simulink model "problem1"  (R2020a)
settings: Solver=VariableStepAuto  StartTime=0.0  StopTime=10.0  RelTol=1e-3
values from neighbouring files (symbols this model uses):
  b = 50.0    [problem_1data.sldd]
  K1 = 50.0    [problem_1data.sldd]
  K12 = 500.0    [problem_1data.sldd]
  M1 = 100.0    [problem_1data.sldd]
  M2 = 5.0    [problem_1data.sldd]
settings Model: Creator=USER  LastModifiedBy=USER

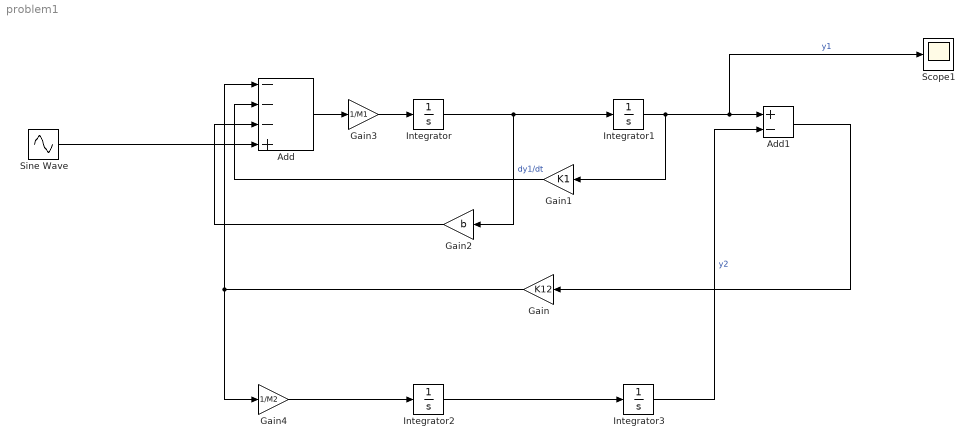
== system problem1 ==
  Add : Sum  Inputs=---+
  Add1 : Sum  Inputs=+-
  Gain : Gain  Gain=K12
  Gain1 : Gain  Gain=K1
  Gain2 : Gain  Gain=b
  Gain3 : Gain  Gain=1/M1
  Gain4 : Gain  Gain=1/M2
  Integrator{,1..3} (4 alike) : Integrator
  Scope1 : Scope
  Sine Wave : Sin  Amplitude=2  Frequency=10  SampleTime=0
  wires:
  Sine Wave/1 -> Add/4
  Add/1 -> Gain3/1
  Gain3/1 -> Integrator/1
  Integrator/1 -> Gain2/1, Integrator1/1  "dy1/dt"
  Gain2/1 -> Add/3
  Gain/1 -> Gain4/1, Add/1
  Add1/1 -> Gain/1
  Gain1/1 -> Add/2
  Integrator3/1 -> Add1/2  "y2"
  Integrator2/1 -> Integrator3/1
  Gain4/1 -> Integrator2/1
  Integrator1/1 -> Gain1/1, Scope1/1, Add1/1  "y1"
